simulink model "simple"  (R2021a)
settings: Solver=FixedStepDiscrete  StartTime=0.0  StopTime=10.0  FixedStep=1.0  RelTol=1e-3
settings Model: EnablePacing=on  PacingRate=0.500000  Creator=yangy  LastModifiedBy=yangy
settings DataIOCC: ExternalInput=port.getElement(1),port.getElement(2)
settings OptimizationCC: DefaultParameterBehavior=Inlined  EnhancedBackFolding=on  PassReuseOutputArgsAs=Individual arguments  ZeroExternalMemoryAtStartup=off  ZeroInternalMemoryAtStartup=off  OptimizeBlockOrder=speed  DifferentSizesBufferReuse=on  OptimizationCustomize=off  EfficientTunableParamExpr=on
settings DebuggingCC: ParameterTunabilityLossMsg=error
settings SFSimCC: MATLABDynamicMemAlloc=off
settings RTWCC: SystemTargetFile=ert.tlc  TemplateMakefile=ert_default_tmf
settings CodeAppCC: ForceParamTrailComments=on  IgnoreCustomStorageClasses=off  OperatorAnnotations=on  SimulinkDataObjDesc=on  SFDataObjDesc=on  InsertBlockDesc=on
settings ERTTargetCC: TargetLangStandard=C99 (ISO)  GenerateSampleERTMain=on  InlinedParameterPlacement=NonHierarchical  ERTCustomFileTemplate=example_file_process.tlc
settings ConfigComp: DVMaxProcessTime=10  DVMaxTestCaseSteps=10  DVTestSuiteOptimization=Auto  DVDetectOutOfBounds=on

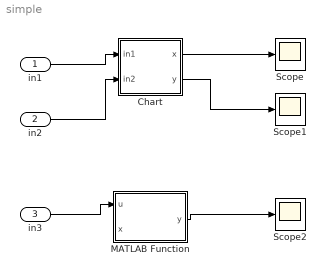
== system simple ==
  in1 : Inport  OutDataTypeStr=double
  in2 : Inport  Port=2  OutDataTypeStr=double
  in3 : Inport  Port=3  OutDataTypeStr=double
  Chart : Stateflow chart  TreatAsAtomicUnit=on
  MATLAB Function : MATLAB Function  TreatAsAtomicUnit=on
  Scope : Scope
  Scope1 : Scope
  Scope2 : Scope
  wires:
  Chart/1(x) -> Scope/1
  Chart/2(y) -> Scope1/1
  in1/1 -> Chart/1(in1)
  in2/1 -> Chart/2(in2)
  MATLAB Function/1(y) -> Scope2/1
  in3/1 -> MATLAB Function/1(u)

== matlab function simple/MATLAB Function ==
  data: u input; y output; x input
function y = fcn(u, x)

y = u;

== stateflow chart simple/Chart ==
  state p1 [parallel]
    settings: executionOrder=1
    state a
      exit:x=10;
    state b
    state c
      entry:x=0;
      state c1
      state c2
      (default) -> c1
      c1 -> c2 : {e;}
      c2 -> c1
    (default) -> p1.a : {x=in1;y=in2;}
    p1.a -> p1.b : e[x==10]{x=x+1;}
    c -> p1.a : e[x==0]{x=0;e;}
    p1.b -> (junction 10) : [x<100]{x=x+1;}
    (junction 10) -> (junction 11) [order 1] : [x<100]{x=x+10;}
    (junction 10) -> (junction 12) [order 2] : [y==0]{y=y+1;}
    (junction 11) -> c : [x==1]{y=y+10;x=x-1;}
    (junction 12) -> c : [y==1]{x=0;}
  state p2 [parallel]
    settings: executionOrder=2
    state a
    state b
    (default) -> p2.a
    p2.a -> p2.b : [x<100]{e;}
    p2.b -> p2.a
  data: x output double =0; y output double =0; in1 input double; in2 input double
  events: e local FUNCTION_CALL_EVENT
